simulink model "DataProcessingSim"  (R2024a)
settings: Solver=VariableStepAuto  StartTime=0.0  StopTime=470000  RelTol=1e-3
libraries: cstblocks x2
settings Model: Creator=ijd9015  LastModifiedBy=ijd9015

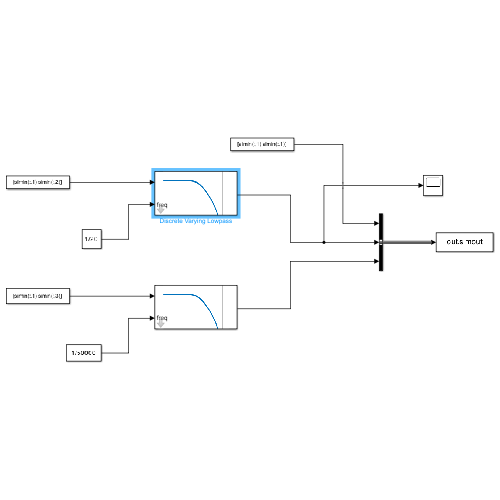
[thumbnail: Simulink's stored preview of the top-level diagram]
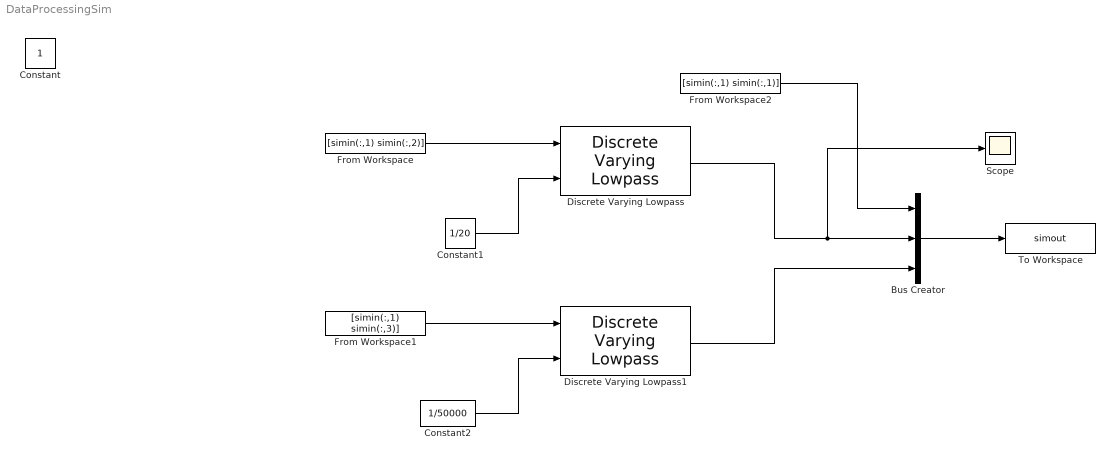
== system DataProcessingSim ==
  Bus Creator : BusCreator  Inputs=3
  Constant1 : Constant  Value=1/20
  Constant2 : Constant  Value=1/50000
  Discrete Varying Lowpass : cstblocks/Linear Parameter Varying/Discrete Varying Lowpass  N=5  w0=0  Ts=10
  Discrete Varying Lowpass1 : cstblocks/Linear Parameter Varying/Discrete Varying Lowpass  N=100  w0=0  Ts=10
  From Workspace : FromWorkspace  VariableName=[simin(:,1) simin(:,2)]  SampleTime=10
  From Workspace1 : FromWorkspace  VariableName=[simin(:,1) simin(:,3)]  SampleTime=10
  From Workspace2 : FromWorkspace  VariableName=[simin(:,1) simin(:,1)]  SampleTime=10
  Scope : Scope
  To Workspace : ToWorkspace  VariableName=simout  SampleTime=-1
      settings: Save2DSignal=2-D array (concatenate along first dimension)
  Constant : Constant  IOType=siggen
  wires:
  Constant1/1 -> Discrete Varying Lowpass/2
  From Workspace/1 -> Discrete Varying Lowpass/1
  Constant2/1 -> Discrete Varying Lowpass1/2
  From Workspace1/1 -> Discrete Varying Lowpass1/1
  Bus Creator/1 -> To Workspace/1
  Discrete Varying Lowpass1/1 -> Bus Creator/3
  Discrete Varying Lowpass/1 -> Scope/1, Bus Creator/2
  From Workspace2/1 -> Bus Creator/1
